simulink model "five_pole_pi_test"  (R2025b)
settings: Solver=VariableStepAuto  StartTime=0.0  StopTime=30  RelTol=1e-3
model workspace (MAT data in the model file):
  C_i = -1358.9
  J_i = -1653.3
  J_p = 75.1522
  Ki = 13194
  Kp = 2976.5
  alpha = 17.4520069808
  beta = 0.0026
  l_eff = 0.4992
  omega_n = 4.4308
settings Model: Creator=clee1  LastModifiedBy=kyue
settings SolverCC: AlgebraicLoopSolver=TrustRegion
settings DebuggingCC: UnconnectedInputMsg=warning  UnconnectedOutputMsg=warning  UnconnectedLineMsg=warning
settings ModelReferenceCC: EnableRefExpFcnMdlSchedulingChecks=on
settings RTWCC: GPUComputeCapability=3.5

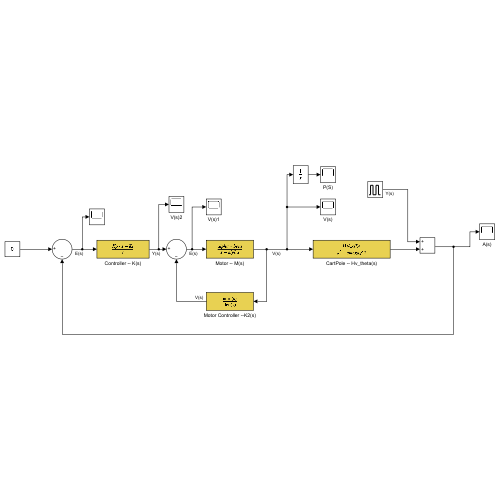
[thumbnail: Simulink's stored preview of the top-level diagram]
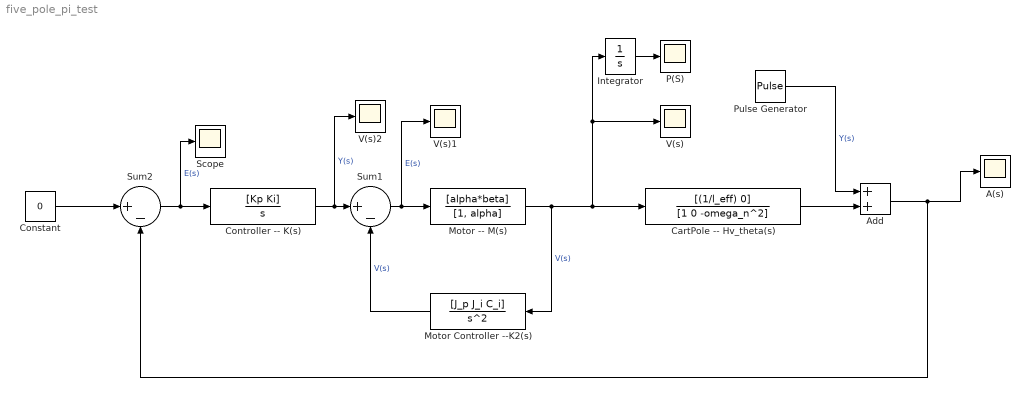
== system five_pole_pi_test ==
  A(s) : Scope
      settings: ActiveDisplayYMinimum=-1.5933343260607908  ActiveDisplayYMaximum=1.3322422833185312
  Add : Sum
  "CartPole -- Hv_theta(s)" : TransferFcn  Numerator=[(1/l_eff) 0]  Denominator=[1 0 -omega_n^2]  ContinuousStateAttributes="\"Controller\""
  Constant : Constant  Value=0
  "Controller -- K(s)" : TransferFcn  Numerator=[Kp Ki]  Denominator=[1 0]  ContinuousStateAttributes="\"Controller\""
  Integrator : Integrator
  "Motor -- M(s)" : TransferFcn  Numerator=[alpha*beta]  Denominator=[1, alpha]  ContinuousStateAttributes="\"Controller\""
  Motor Controller --K2(s) : TransferFcn  Numerator=[J_p J_i C_i]  Denominator=[1 0 0 ]  ContinuousStateAttributes="\"Controller\""
  P(S) : Scope
      settings: ActiveDisplayYMinimum=-60.804609133471267  ActiveDisplayYMaximum=21.782554078648378  DataLoggingVariableName=ScopeData5
  Pulse Generator : DiscretePulseGenerator  PulseType=Time based  Amplitude=.5  Period=7  PulseWidth=.1
  Scope : Scope
      settings: DataLoggingVariableName=ScopeData4
  Sum1 : Sum  Inputs=|+-
  Sum2 : Sum  Inputs=|+-
  V(s) : Scope
      settings: ActiveDisplayYMinimum=-0.9651191045310743  ActiveDisplayYMaximum=0.42752289608572841
  V(s)1 : Scope
      settings: ActiveDisplayYMinimum=-0.4306163769511912  ActiveDisplayYMaximum=0.20116990303484833  DataLoggingVariableName=ScopeData2
  V(s)2 : Scope
      settings: ActiveDisplayYMinimum=-0.4306163769511912  ActiveDisplayYMaximum=0.20116990303484833  DataLoggingVariableName=ScopeData3
  wires:
  Sum2/1 -> Scope/1, "Controller -- K(s)"/1  "E(s)"
  "Motor -- M(s)"/1 -> Motor Controller --K2(s)/1, Integrator/1, V(s)/1, "CartPole -- Hv_theta(s)"/1  "V(s)"
  "CartPole -- Hv_theta(s)"/1 -> Add/2
  Constant/1 -> Sum2/1
  Add/1 -> Sum2/2, A(s)/1
  Pulse Generator/1 -> Add/1  "Y(s)"
  Integrator/1 -> P(S)/1
  "Controller -- K(s)"/1 -> V(s)2/1, Sum1/1  "Y(s)"
  Sum1/1 -> V(s)1/1, "Motor -- M(s)"/1  "E(s)"
  Motor Controller --K2(s)/1 -> Sum1/2  "V(s)"
